simulink model "gm_HDLFreqUpshift_vs"  (R2024a)
settings: Solver=FixedStepDiscrete  StartTime=0.0  StopTime=stopTime  RelTol=1e-3
undefined symbols (not defined in the file or in its folder): clk, clk_enable, fs, reset_x
libraries: dspsrcs4 x3, simulink x2, HDL_ieee_8021513 x2, whdlutilities x1, vivadosimlib x1
settings Model: Creator=cotti  LastModifiedBy=cotti
settings OptimizationCC: BlockReduction=off  ConditionallyExecuteInputs=off  DefaultParameterBehavior=Inlined  InheritOutputTypeSmallerThanSingle=on
settings DebuggingCC: AlgebraicLoopMsg=error  ArtificialAlgebraicLoopMsg=error  InheritedTsInSrcMsg=none  SingleTaskRateTransMsg=error  UnconnectedInputMsg=warning  UnconnectedOutputMsg=warning  UnconnectedLineMsg=warning
settings HardwareCC: ProdBitPerPointer=32  ProdBitPerSizeT=32  ProdBitPerPtrDiffT=32  ProdLargestAtomicFloat=None  ProdIntDivRoundTo=Undefined  ProdEndianess=Unspecified  ProdWordSize=32  ProdHWDeviceType=ASIC/FPGA->ASIC/FPGA  TargetBitPerLong=64  TargetBitPerPointer=64  TargetBitPerSizeT=64  TargetBitPerPtrDiffT=64  TargetLongLongMode=on  TargetIntDivRoundTo=Zero  TargetEndianess=LittleEndian  TargetWordSize=64  TargetHWDeviceType=Custom Processor->MATLAB Host Computer  ProdEqTarget=off

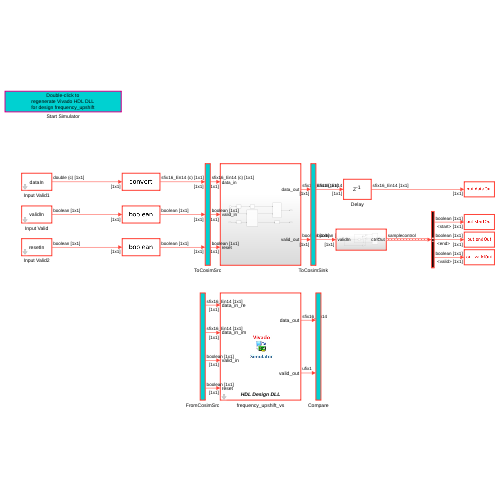
[thumbnail: Simulink's stored preview of the top-level diagram]
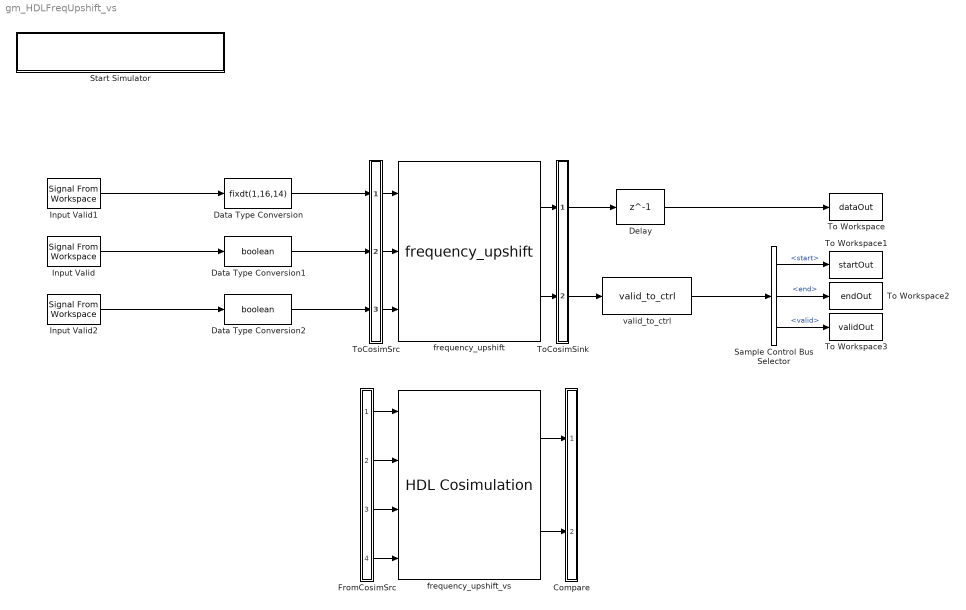
== system gm_HDLFreqUpshift_vs ==
  Compare : Subsystem
      mask Display: disp('')
  Data Type Conversion : DataTypeConversion  OutDataTypeStr=fixdt(1,16,14)  SaturateOnIntegerOverflow=off  RndMeth=Floor
  Data Type Conversion1 : DataTypeConversion  OutDataTypeStr=boolean  SaturateOnIntegerOverflow=off  RndMeth=Floor
  Data Type Conversion2 : DataTypeConversion  OutDataTypeStr=boolean  SaturateOnIntegerOverflow=off  RndMeth=Floor
  Delay : Delay  DelayLength=1  InitialCondition=0  UseCircularBuffer=on
  FromCosimSrc : Subsystem
      mask Display: disp('')
  Input Valid : dspsrcs4/Signal From Workspace  X=validIn  Ts=1/fs  nsamps=1  OutputAfterFinalValue=Setting to zero  ignoreOrWarnInputAndFrameLengths=off  OutputFrames=off
  Input Valid1 : dspsrcs4/Signal From Workspace  X=dataIn  Ts=1/fs  nsamps=1  OutputAfterFinalValue=Setting to zero  ignoreOrWarnInputAndFrameLengths=off  OutputFrames=off
  Input Valid2 : dspsrcs4/Signal From Workspace  X=resetIn  Ts=1/fs  nsamps=1  OutputAfterFinalValue=Setting to zero  ignoreOrWarnInputAndFrameLengths=off  OutputFrames=off
  Sample Control Bus Selector : whdlutilities/Sample Control Bus Selector  OutputSignals=start,end,valid
  Start Simulator : Subsystem
      settings: OpenFcn=|
      | cosimDirName = pwd;
      | cd 'hdl_prj/hdlsrc/HDLFreqUpshift';
      | [s,r] = system('vivado -mode batch -source gm_HDLFreqUpshift_vs.tcl','-echo');
      | cd (cosimDirName);
      | clear cosimDirName;
      | if s
      |    error('Failed to create Vivado HDL design DLL using script gm_HDLFreqUpshift_vs.tcl.');
      | end
      mask Display: disp('Double-click to\nregenerate Vivado HDL DLL\nfor design frequency_upshift')
  To Workspace : ToWorkspace  VariableName=dataOut  SampleTime=1/fs
      settings: Save2DSignal=2-D array (concatenate along first dimension)
  To Workspace1 : ToWorkspace  VariableName=startOut  SampleTime=1/fs
      settings: Save2DSignal=2-D array (concatenate along first dimension)
  To Workspace2 : ToWorkspace  VariableName=endOut  SampleTime=1/fs
      settings: Save2DSignal=2-D array (concatenate along first dimension)
  To Workspace3 : ToWorkspace  VariableName=validOut  SampleTime=1/fs
      settings: Save2DSignal=2-D array (concatenate along first dimension)
  ToCosimSink : Subsystem
      mask Display: disp('')
  ToCosimSrc : Subsystem
      mask Display: disp('')
  frequency_upshift : HDL_ieee_8021513/frequency_upshift  SystemSampleTime=-1  VariantActivationTime=update diagram  AllowFlexibleInterface=on  Latency=0  AutoFrameSizeCalculation=off
      settings: SourceProductName=HDL IEEE 8021513
  frequency_upshift_vs : vivadosimlib/HDL Cosimulation  PortPaths=/frequency_upshift/data_in_re;/frequency_upshift/data_in_im;/frequency_upshift/valid_in;/frequency_upshift/reset;/frequency_upshift/data_out;/frequency_upshift/valid_out  PortModes=[1 1 1 1 2 2 ]  PortTimes=[-1 -1 -1 -1 1.0000000000000000209225608301284726753266340892878361046314239502e-08 1.0000000000000000209225608301284726753266340892878361046314239502e-08 ]  PortSigns=[-1 -1 -1 -1 1 0 ]  PortFracLengths=[0,0,0,0,14,0]  PortWordLengths=[-1,-1,-1,-1,16,1]  PortHDLWordSizes=[16,16,1,1,16,1]  CommLocal=on  CommSharedMemory=on  CommPortNumber=4449  CommShowInfo=on  ClockPaths=clk;clk_enable;reset_x;  ClockModes=[2 4 3]  ClockTimes=[1e-08 3.7e-08 2.7e-08]  TclPostSimCommand="puts \"done\""  TimingMode=ns  TimingScaleFactor=1000000000  idxCellArray={'UNUSED_VAR'}  CosimBypass=Full Simulation  AllowDirectFeedthrough=on  ProductName=EDA Simulator Link VS  RunAutoTimescale=off  HdlClocks=0  PreRunTime=40  PreRunTimeUnit=ns
  valid_to_ctrl : HDL_ieee_8021513/valid_to_ctrl  SystemSampleTime=-1  VariantActivationTime=update diagram  AllowFlexibleInterface=on  Latency=0  AutoFrameSizeCalculation=off
      settings: SourceProductName=HDL IEEE 8021513
  wires:
  valid_to_ctrl/1 -> Sample Control Bus Selector/1
  Sample Control Bus Selector/1 -> To Workspace1/1  "<start>"
  Sample Control Bus Selector/2 -> To Workspace2/1  "<end>"
  Sample Control Bus Selector/3 -> To Workspace3/1  "<valid>"
  Delay/1 -> To Workspace/1
  Input Valid/1 -> Data Type Conversion1/1
  Input Valid1/1 -> Data Type Conversion/1
  Input Valid2/1 -> Data Type Conversion2/1
  ToCosimSrc/1(out1) -> frequency_upshift/1
  ToCosimSrc/2(out2) -> frequency_upshift/2
  ToCosimSrc/3(out3) -> frequency_upshift/3
  frequency_upshift/1 -> ToCosimSink/1(in1)
  frequency_upshift/2 -> ToCosimSink/2(in2)
  Data Type Conversion/1 -> ToCosimSrc/1(in1)
  Data Type Conversion1/1 -> ToCosimSrc/2(in2)
  Data Type Conversion2/1 -> ToCosimSrc/3(in3)
  ToCosimSink/1(out1) -> Delay/1
  ToCosimSink/2(out2) -> valid_to_ctrl/1
  FromCosimSrc/1(out1) -> frequency_upshift_vs/1
  FromCosimSrc/2(out2) -> frequency_upshift_vs/2
  FromCosimSrc/3(out3) -> frequency_upshift_vs/3
  FromCosimSrc/4(out4) -> frequency_upshift_vs/4
  frequency_upshift_vs/1 -> Compare/1(in1)
  frequency_upshift_vs/2 -> Compare/2(in2)

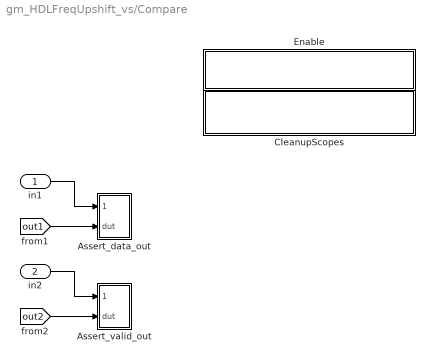
== system gm_HDLFreqUpshift_vs/Compare ==
  in1 : Inport
  in2 : Inport  Port=2
  Assert_data_out : Subsystem
      settings: LibrarySourceBlock=hdlmdlgenlib/AssertEq
  Assert_valid_out : Subsystem
      settings: LibrarySourceBlock=hdlmdlgenlib/AssertEq
  CleanupScopes : Subsystem
      settings: OpenFcn=|
      | blkName = gcb; %self block
      | idx = regexp(blkName, '/CleanupScopes$', 'once');
      | blkParent = blkName(1:idx-1);
      | blks=find_system(blkParent, 'LookUnderMasks', 'all','blocktype', 'Scope');
      | for itr = 1:length(blks)
      | 	 hScopeCfg = get_param(blks{itr},'ScopeConfiguration');
      | 	 hScopeCfg.Visible = ~ hScopeCfg.Visible;
      | end
      | drawnow;
      mask Display: fprintf(message('hdlcoder:cosim:vnl_dblclick').getString());
  Enable : Subsystem
      settings: OpenFcn=|
      | blkName = gcb;
      | idx = regexp(blkName, '/Enable$', 'once');
      | blkParent = blkName(1:idx-1);
      | blks=find_system(blkParent, 'LookUnderMasks', 'all','blocktype', 'Assertion');
      | e = get_param(blks{1}, 'Enabled');
      | if strcmp(e, 'on'), f= 'off';, else, f = 'on';, end
      | for ii=1:length(blks), set_param(blks{ii}, 'Enabled', f);, end
      | set_param(gcb, 'MaskDisplay',['fprintf(message(''hdlcoder:cosim:vnl_dblclick_assertions'',','''',upper(e),'''',').getString())']);
      mask Display: fprintf(message('hdlcoder:cosim:vnl_dblclick_assertions','OFF').getString());
  wires:
  [out2] -> Assert_valid_out/2(dut)
  in2/1 -> Assert_valid_out/1(cosim)
  [out1] -> Assert_data_out/2(dut)
  in1/1 -> Assert_data_out/1(cosim)

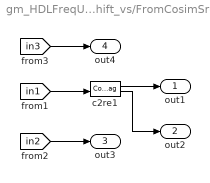
== system gm_HDLFreqUpshift_vs/FromCosimSrc ==
  c2re1 : ComplexToRealImag
  out1 : Outport
  out2 : Outport  Port=2
  out3 : Outport  Port=3
  out4 : Outport  Port=4
  wires:
  c2re1/2 -> out2/1
  [in2] -> out3/1
  c2re1/1 -> out1/1
  [in1] -> c2re1/1
  [in3] -> out4/1

== system gm_HDLFreqUpshift_vs/Start Simulator ==

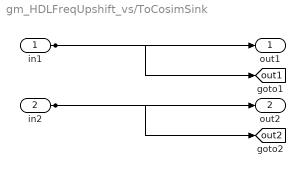
== system gm_HDLFreqUpshift_vs/ToCosimSink ==
  in1 : Inport
  in2 : Inport  Port=2
  out1 : Outport
  out2 : Outport  Port=2
  tag scope: out1=global, out2=global
  wires:
  in1/1 -> out1/1, [out1]
  in2/1 -> out2/1, [out2]

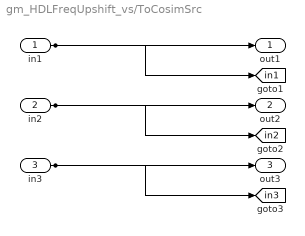
== system gm_HDLFreqUpshift_vs/ToCosimSrc ==
  in1 : Inport
  in2 : Inport  Port=2
  in3 : Inport  Port=3
  out1 : Outport
  out2 : Outport  Port=2
  out3 : Outport  Port=3
  tag scope: in1=global, in2=global, in3=global
  wires:
  in1/1 -> out1/1, [in1]
  in2/1 -> out2/1, [in2]
  in3/1 -> out3/1, [in3]

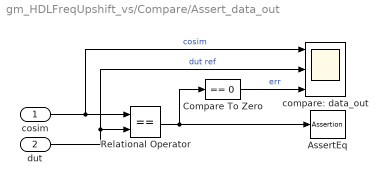
== system gm_HDLFreqUpshift_vs/Compare/Assert_data_out ==
  cosim : Inport
  dut : Inport  Port=2
  AssertEq : Assertion
  Compare To Zero : simulink/Logic and Bit Operations/Compare To Zero  relop===  OutDataTypeStr=boolean
  Relational Operator : RelationalOperator  Operator===  OutDataTypeStr=boolean  InputSameDT=off
  compare: data_out : Scope  NumInputPorts=3
  wires:
  Compare To Zero/1 -> compare: data_out/3  "err"
  Relational Operator/1 -> Compare To Zero/1, AssertEq/1
  cosim/1 -> compare: data_out/1, Relational Operator/1  "cosim"
  dut/1 -> compare: data_out/2, Relational Operator/2  "dut ref"

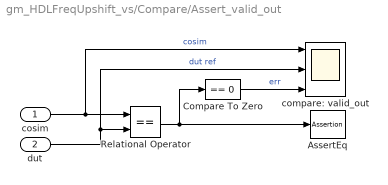
== system gm_HDLFreqUpshift_vs/Compare/Assert_valid_out ==
  cosim : Inport
  dut : Inport  Port=2
  AssertEq : Assertion
  Compare To Zero : simulink/Logic and Bit Operations/Compare To Zero  relop===  OutDataTypeStr=boolean
  Relational Operator : RelationalOperator  Operator===  OutDataTypeStr=boolean  InputSameDT=off
  compare: valid_out : Scope  NumInputPorts=3
  wires:
  Compare To Zero/1 -> compare: valid_out/3  "err"
  Relational Operator/1 -> Compare To Zero/1, AssertEq/1
  cosim/1 -> compare: valid_out/1, Relational Operator/1  "cosim"
  dut/1 -> compare: valid_out/2, Relational Operator/2  "dut ref"

== system gm_HDLFreqUpshift_vs/Compare/CleanupScopes ==

== system gm_HDLFreqUpshift_vs/Compare/Enable ==
